simulink model "energybasedHosseinEd.old"  (R2020a)
settings: Solver=FixedStepDiscrete  StartTime=0.0  StopTime=Tsim  FixedStep=Ts  RelTol=1e-3
values from neighbouring files (symbols this model uses):
  EN_RATIO_LIMIT = param.EN_RATIO_LIMIT    [energybased.m]    (also in energybased.old.m = 0.3)
  En_Threshold = param.En_Threshold    [energybased.m]    (also in run.m = 2e-06; thresholdSet.m = 1e-08)
  M = ones(1,m)    [energybased.m]    (also in energybased.old.m; run.m)
  m = floor(m)    [energybased.m]    (also in energybased.old.m = ceil(Freq_stop0/Test.TPE)*Test.TPE/fT-m1; run.m)
  m1 = ceil(Freq_start0/fT)    [energybased.m]    (also in energybased.old.m)
  n_tpe = param.n_tpe    [energybased.m]    (also in energybased.old.m = 20; run.m = echdParam.n_tpe)
  nd_mean = round((1/Test.SF)/Ts)    [energybased.m]    (also in energybased.old.m; run.m = round((1/samplingFreq)/samplingInterval))
  num_delay = round((1/Test.SF)/Ts/2) * 5    [energybased.m]    (also in energybased.old.m; run.m = round((1/samplingFreq)/samplingInterval/2) * 5)
  TP_P0 = 1e1*eye(2*n_tpe)    [energybased.m]    (also in energybased.old.m; run.m)
  TP_PHI = zeros(2*n_tpe, 1)    [energybased.m]    (also in energybased.old.m; run.m)
  TP_Q = TP_R*lambda    [energybased.m]    (also in energybased.old.m; run.m)
  TP_q0 = zeros(2*n_tpe, 1)    [energybased.m]    (also in energybased.old.m; run.m)
  TP_R = 8.539750000056574E-6    (= 8.53975000006e-06)    [energybased.m]    (also in energybased.old.m; run.m)
  Ts = 1/properties.sampling    [energybased.m]    (also in energybased.old.m = 1/sampling)
  w_BOL = 1    [energybased.m]    (also in run.m; thresholdSet.m)
undefined symbols (not defined in the file or in its folder): Test
libraries: simulink x1
settings Model: Creator=Yudi Wang  LastModifiedBy=mhoss
settings DataIOCC: ReturnWorkspaceOutputs=off
settings DebuggingCC: ReadBeforeWriteMsg=DisableAll  WriteAfterWriteMsg=DisableAll  WriteAfterReadMsg=DisableAll  MultiTaskDSMMsg=none  ArithmeticOperatorsInVariantConditions=warning
settings ModelReferenceCC: UpdateModelReferenceTargets=IfOutOfDate
settings SFSimCC: SFSimEcho=off  SimUseLocalCustomCode=off  CustomCodeUndefinedFunction=UseInterfaceOnly
settings RTWCC: RTWUseLocalCustomCode=off

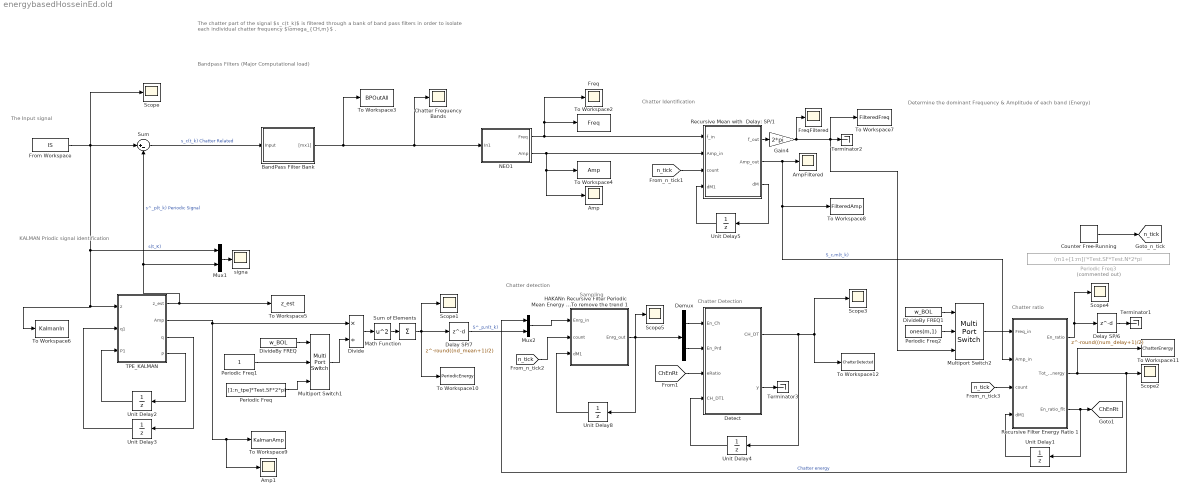
== system energybasedHosseinEd.old ==
  note: The chatter part of the signal $s_c(t_k)$ is filtered through a bank of band pass filters in order to isolate each individual chatter frequency $\omega_{CH,m}$ .
  note: Chatter Identification
  note: Chatter Detection
  note: Bandpass Filters
      | (Major Computational load)
  note: KALMAN
      | Priodic signal identification
  note: Chatter detection
  note: Chatter ratio
  note: The Input signal
  note: Determine the dominant Frequency & Amplitude of each band
      | (Energy)
  note: Sampling
  Amp : Scope
  Amp1 : Scope
  AmpFiltered : Scope
  BandPass Filter Bank : Subsystem
  Chatter Frequency Bands : Scope
  Counter Free-Running : simulink/Sources/Counter Free-Running  NumBits=32  tsamp=Ts
  Delay SP/6 : Delay  DelayLength=round((num_delay+1)/2)
  Delay SP/7 : Delay  DelayLength=round((nd_mean+1)/2)
  Demux : Demux  Outputs=2
  Detect : MATLAB Function  TreatAsAtomicUnit=on
  Divide : Product  Inputs=*/
  DivideBy FREQ : Constant  Value=w_BOL
  DivideBy FREQ1 : Constant  Value=w_BOL
  Freq : Scope
  FreqFiltered : Scope
  From Workspace : FromWorkspace  VariableName=IS  SampleTime=Ts  OutputAfterFinalValue=Setting to zero
  Gain4 : Gain  Gain=2*pi
  HAKANn Recursive Filter Periodic Mean Energy To remove the trend 1 : MATLAB Function  TreatAsAtomicUnit=on
  Math Function : Math  Operator=square  SignedPower=on  SaturateOnIntegerOverflow=on
  Multiport Switch1 : MultiPortSwitch  Inputs=2
  Multiport Switch2 : MultiPortSwitch  Inputs=2
  Mux1 : Mux  Inputs=2
  Mux2 : Mux  Inputs=2
  NEO1 : Subsystem
  Periodic Freq : Constant  Value=[1:n_tpe]*Test.SF*2*pi
  Periodic Freq1 : Constant
  Periodic Freq2 : Constant  Value=ones(m,1)
  Periodic Freq3 : Constant  Commented=on  Value=(m1+[1:m])'*Test.SF*Test.N*2*pi
  Recursive Mean with  Delay: SP/1 : MATLAB Function  TreatAsAtomicUnit=on
  Recursive Filter Energy Ratio 1 : MATLAB Function  TreatAsAtomicUnit=on
  Scope{,1..5} (6 alike) : Scope
  Sum : Sum  Inputs=|+-
  Sum of Elements : Sum  Inputs=+
  TPE_KALMAN : MATLAB Function  TreatAsAtomicUnit=on
  Terminator1 : Terminator
  Terminator2 : Terminator
  Terminator3 : Terminator
  To Workspace10 : ToWorkspace  VariableName=PeriodicEnergy  SaveFormat=Structure With Time  SampleTime=-1
  To Workspace11 : ToWorkspace  VariableName=ChatterEnergy  SaveFormat=Structure With Time  SampleTime=-1
  To Workspace12 : ToWorkspace  VariableName=ChatterDetected  SaveFormat=Structure With Time  SampleTime=-1
  To Workspace2 : ToWorkspace  VariableName=Freq  SaveFormat=Structure With Time  SampleTime=-1
  To Workspace3 : ToWorkspace  VariableName=BPOutAll  SaveFormat=Structure With Time  SampleTime=-1
  To Workspace4 : ToWorkspace  VariableName=Amp  SaveFormat=Structure With Time  SampleTime=-1
  To Workspace5 : ToWorkspace  VariableName=z_est  SaveFormat=Structure With Time  SampleTime=-1
  To Workspace6 : ToWorkspace  VariableName=KalmanIn  SaveFormat=Structure With Time  SampleTime=-1
  To Workspace7 : ToWorkspace  VariableName=FilteredFreq  SaveFormat=Structure With Time  SampleTime=-1
  To Workspace8 : ToWorkspace  VariableName=FilteredAmp  SaveFormat=Structure With Time  SampleTime=-1
  To Workspace9 : ToWorkspace  VariableName=KalmanAmp  SaveFormat=Structure With Time  SampleTime=-1
  Unit Delay1 : UnitDelay  SampleTime=Ts  HasFrameUpgradeWarning=on
  Unit Delay2 : UnitDelay  InitialCondition=TP_P0  SampleTime=-1  HasFrameUpgradeWarning=on
  Unit Delay3 : UnitDelay  InitialCondition=TP_q0  SampleTime=-1  HasFrameUpgradeWarning=on
  Unit Delay4 : UnitDelay  SampleTime=-1  HasFrameUpgradeWarning=on
  Unit Delay5 : UnitDelay  SampleTime=-1  HasFrameUpgradeWarning=on
  Unit Delay8 : UnitDelay  SampleTime=Ts  HasFrameUpgradeWarning=on
  signa : Scope
  tag scope: ChEnRt=global, n_tick=global
  wires:
  Mux1/1 -> signa/1
  HAKANn Recursive Filter Periodic Mean Energy To remove the trend 1/1(Enrg_out) -> Demux/1, Scope5/1, Unit Delay8/1
  Sum/1 -> BandPass Filter Bank/1(Input)  "s_c(t_k) Chatter Related"
  Multiport Switch2/1 -> Recursive Filter Energy Ratio 1/1(Freq_in)
  Periodic Freq1/1 -> Multiport Switch1/2
  TPE_KALMAN/1(z_est) -> Mux1/2, Sum/2, To Workspace5/1  "s^_p(t_k) Periodic Signal"
  Math Function/1 -> Sum of Elements/1
  TPE_KALMAN/4(P) -> Unit Delay2/1
  BandPass Filter Bank/1("[mx1]") -> To Workspace3/1, NEO1/1(In1), Chatter Frequency Bands/1
  Detect/2(y) -> Terminator3/1
  [n_tick] -> HAKANn Recursive Filter Periodic Mean Energy To remove the trend 1/2(count)
  TPE_KALMAN/2(Amp) -> Divide/1, Amp1/1, To Workspace9/1
  Counter Free-Running/1 -> [n_tick]
  NEO1/1(Freq) -> Recursive Mean with  Delay: SP/1/1(f_in), Freq/1, To Workspace2/1
  Recursive Filter Energy Ratio 1/3(En_ratio_flt) -> [ChEnRt], Unit Delay1/1
  Detect/1(CH_DT) -> Unit Delay4/1, To Workspace12/1, Scope3/1
  [n_tick] -> Recursive Mean with  Delay: SP/1/3(count)
  Recursive Filter Energy Ratio 1/2(Tot_CH_Energy) -> To Workspace11/1, Mux2/1, Scope2/1  "Chatter energy"
  Periodic Freq2/1 -> Multiport Switch2/2
  Recursive Mean with  Delay: SP/1/3(dM) -> Unit Delay5/1
  Unit Delay4/1 -> Detect/4(CH_DT1)
  Recursive Mean with  Delay: SP/1/1(f_out) -> Gain4/1
  Divide/1 -> Math Function/1
  NEO1/2(Amp) -> Recursive Mean with  Delay: SP/1/2(Amp_in), Amp/1, To Workspace4/1
  Periodic Freq/1 -> Multiport Switch1/3
  From Workspace/1 -> Scope/1, To Workspace6/1, TPE_KALMAN/1(z), Mux1/1, Sum/1  "s(t_K)"
  Unit Delay8/1 -> HAKANn Recursive Filter Periodic Mean Energy To remove the trend 1/3(dM1)
  Unit Delay5/1 -> Recursive Mean with  Delay: SP/1/4(dM1)
  [n_tick] -> Recursive Filter Energy Ratio 1/3(count)
  Demux/2 -> Detect/2(En_Prd)
  TPE_KALMAN/3(q) -> Unit Delay3/1
  DivideBy FREQ/1 -> Multiport Switch1/1
  Unit Delay1/1 -> Recursive Filter Energy Ratio 1/4(dM1)
  Gain4/1 -> FreqFiltered/1, Terminator2/1, To Workspace7/1, Multiport Switch2/3
  Multiport Switch1/1 -> Divide/2
  Recursive Filter Energy Ratio 1/1(En_ratio) -> Delay SP/6/1, Scope4/1
  Demux/1 -> Detect/1(En_Ch)
  [ChEnRt] -> Detect/3(eRatio)
  Unit Delay3/1 -> TPE_KALMAN/2(q1)
  Unit Delay2/1 -> TPE_KALMAN/3(P1)
  Mux2/1 -> HAKANn Recursive Filter Periodic Mean Energy To remove the trend 1/1(Enrg_in)
  Sum of Elements/1 -> To Workspace10/1, Delay SP/7/1, Scope1/1
  DivideBy FREQ1/1 -> Multiport Switch2/1
  Recursive Mean with  Delay: SP/1/2(Amp_out) -> Recursive Filter Energy Ratio 1/2(Amp_in), To Workspace8/1, AmpFiltered/1  "S_c,m(t_k)"
  Delay SP/6/1 -> Terminator1/1
  Delay SP/7/1 -> Mux2/2  "S^_p,n(t_k)"

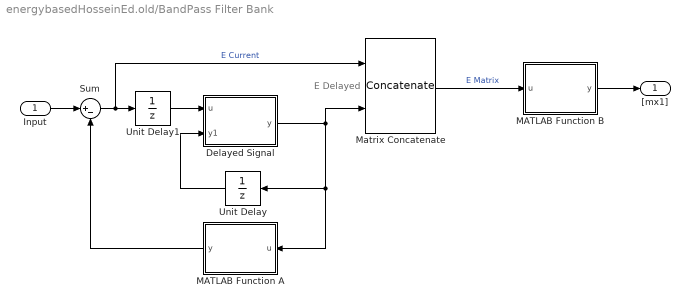
== system energybasedHosseinEd.old/BandPass Filter Bank ==
  note: E Delayed
  Input : Inport
  Delayed Signal : MATLAB Function  TreatAsAtomicUnit=on
  MATLAB Function A : MATLAB Function  TreatAsAtomicUnit=on
  MATLAB Function B : MATLAB Function  TreatAsAtomicUnit=on
  Matrix Concatenate : Concatenate  Mode=Multidimensional array  ConcatenateDimension=2
  Sum : Sum  Inputs=|+-
  Unit Delay : UnitDelay  SampleTime=-1  HasFrameUpgradeWarning=on
  Unit Delay1 : UnitDelay  SampleTime=-1  HasFrameUpgradeWarning=on
  "[mx1]" : Outport  VectorParamsAs1DForOutWhenUnconnected=off
  wires:
  Delayed Signal/1(y) -> Unit Delay/1, MATLAB Function A/1(u), Matrix Concatenate/2
  Unit Delay/1 -> Delayed Signal/2(y1)
  Unit Delay1/1 -> Delayed Signal/1(u)
  Sum/1 -> Unit Delay1/1, Matrix Concatenate/1  "E Current"
  Input/1 -> Sum/1
  MATLAB Function A/1(y) -> Sum/2
  Matrix Concatenate/1 -> MATLAB Function B/1(u)  "E Matrix"
  MATLAB Function B/1(y) -> "[mx1]"/1

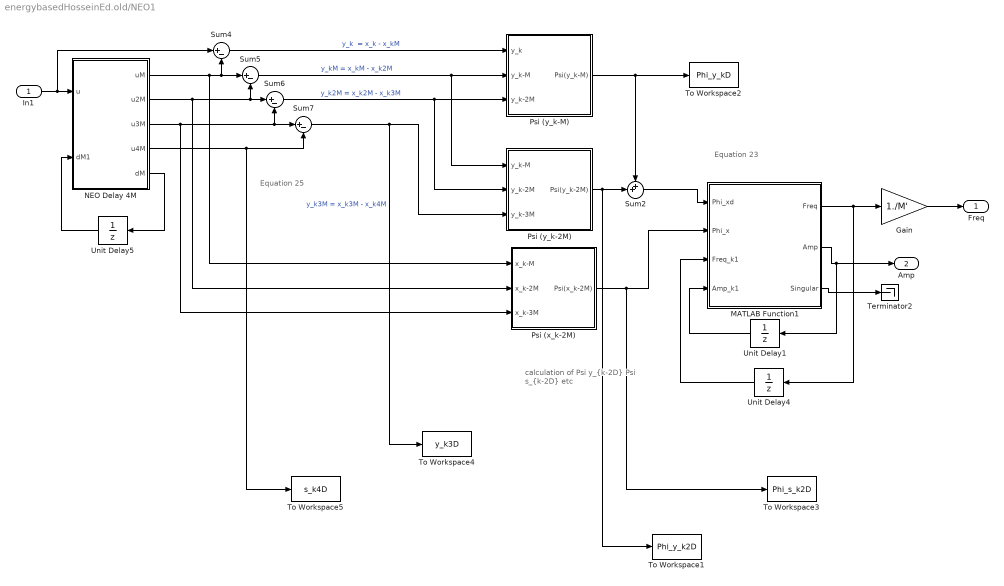
== system energybasedHosseinEd.old/NEO1 ==
  note: calculation of
      | Psi y_{k-2D}
      | Psi s_{k-2D} etc
  note: Equation 23
  note: Equation 25
  In1 : Inport
  Gain : Gain  Gain=1./M'
  MATLAB Function1 : MATLAB Function  TreatAsAtomicUnit=on
  NEO Delay 4M : MATLAB Function  TreatAsAtomicUnit=on
  Psi (x_k-2M) : Subsystem
  Psi (y_k-2M) : Subsystem
  Psi (y_k-M) : Subsystem
  Sum2 : Sum  Inputs=++|
  Sum{4..7} (4 alike) : Sum  Inputs=|+-
  Terminator2 : Terminator
  To Workspace1 : ToWorkspace  VariableName=Phi_y_k2D  SaveFormat=Structure With Time  SampleTime=-1
  To Workspace2 : ToWorkspace  VariableName=Phi_y_kD  SaveFormat=Structure With Time  SampleTime=-1
  To Workspace3 : ToWorkspace  VariableName=Phi_s_k2D  SaveFormat=Structure With Time  SampleTime=-1
  To Workspace4 : ToWorkspace  VariableName=y_k3D  SaveFormat=Structure With Time  SampleTime=-1
  To Workspace5 : ToWorkspace  VariableName=s_k4D  SaveFormat=Structure With Time  SampleTime=-1
  Unit Delay1 : UnitDelay  SampleTime=Ts  HasFrameUpgradeWarning=on
  Unit Delay4 : UnitDelay  SampleTime=Ts  HasFrameUpgradeWarning=on
  Unit Delay5 : UnitDelay  SampleTime=Ts  HasFrameUpgradeWarning=on
  Freq : Outport  VectorParamsAs1DForOutWhenUnconnected=off
  Amp : Outport  Port=2  VectorParamsAs1DForOutWhenUnconnected=off
  wires:
  Sum4/1 -> Psi (y_k-M)/1(y_k)  "y_k  = x_k - x_kM"
  NEO Delay 4M/5(dM) -> Unit Delay5/1
  Unit Delay5/1 -> NEO Delay 4M/2(dM1)
  NEO Delay 4M/1(uM) -> Sum4/2, Sum5/1, Psi (x_k-2M)/1(x_k-M)
  Sum5/1 -> Psi (y_k-M)/2(y_k-M), Psi (y_k-2M)/1(y_k-M)  "y_kM = x_kM - x_k2M"
  NEO Delay 4M/3(u3M) -> Sum6/2, Sum7/1, Psi (x_k-2M)/3(x_k-3M)
  Sum6/1 -> Psi (y_k-M)/3(y_k-2M), Psi (y_k-2M)/2(y_k-2M)  "y_k2M = x_k2M - x_k3M"
  In1/1 -> NEO Delay 4M/1(u), Sum4/1
  Psi (y_k-M)/1(Psi(y_k-M)) -> To Workspace2/1, Sum2/1
  NEO Delay 4M/2(u2M) -> Sum6/1, Sum5/2, Psi (x_k-2M)/2(x_k-2M)
  NEO Delay 4M/4(u4M) -> To Workspace5/1, Sum7/2
  Sum7/1 -> To Workspace4/1, Psi (y_k-2M)/3(y_k-3M)  "y_k3M = x_k3M - x_k4M"
  Psi (y_k-2M)/1(Psi(y_k-2M)) -> To Workspace1/1, Sum2/2
  Unit Delay1/1 -> MATLAB Function1/4(Amp_k1)
  Unit Delay4/1 -> MATLAB Function1/3(Freq_k1)
  MATLAB Function1/1(Freq) -> Unit Delay4/1, Gain/1
  Gain/1 -> Freq/1
  MATLAB Function1/2(Amp) -> Unit Delay1/1, Amp/1
  Psi (x_k-2M)/1(Psi(x_k-2M)) -> To Workspace3/1, MATLAB Function1/2(Phi_x)
  Sum2/1 -> MATLAB Function1/1(Phi_xd)
  MATLAB Function1/3(Singular) -> Terminator2/1

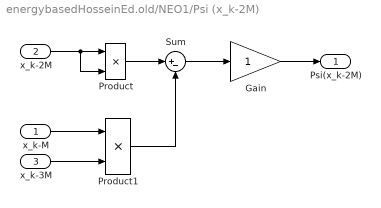
== system energybasedHosseinEd.old/NEO1/Psi (x_k-2M) ==
  x_k-M : Inport
  x_k-2M : Inport  Port=2
  x_k-3M : Inport  Port=3
  Gain : Gain
  Product : Product
  Product1 : Product
  Sum : Sum  Inputs=|+-
  Psi(x_k-2M) : Outport  VectorParamsAs1DForOutWhenUnconnected=off
  wires:
  Product1/1 -> Sum/2
  Sum/1 -> Gain/1
  Gain/1 -> Psi(x_k-2M)/1
  x_k-M/1 -> Product1/1
  x_k-3M/1 -> Product1/2
  Product/1 -> Sum/1
  x_k-2M/1 -> Product/2, Product/1

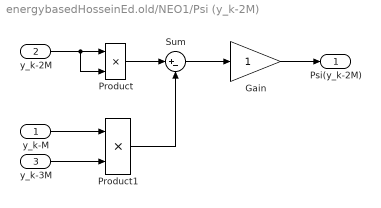
== system energybasedHosseinEd.old/NEO1/Psi (y_k-2M) ==
  y_k-M : Inport
  y_k-2M : Inport  Port=2
  y_k-3M : Inport  Port=3
  Gain : Gain
  Product : Product
  Product1 : Product
  Sum : Sum  Inputs=|+-
  Psi(y_k-2M) : Outport  VectorParamsAs1DForOutWhenUnconnected=off
  wires:
  y_k-2M/1 -> Product/1, Product/2
  Product/1 -> Sum/1
  y_k-3M/1 -> Product1/2
  y_k-M/1 -> Product1/1
  Gain/1 -> Psi(y_k-2M)/1
  Sum/1 -> Gain/1
  Product1/1 -> Sum/2

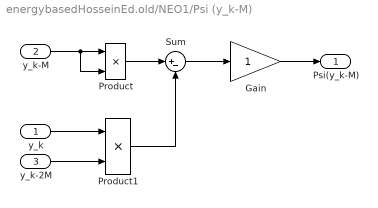
== system energybasedHosseinEd.old/NEO1/Psi (y_k-M) ==
  y_k : Inport
  y_k-M : Inport  Port=2
  y_k-2M : Inport  Port=3
  Gain : Gain
  Product : Product
  Product1 : Product
  Sum : Sum  Inputs=|+-
  Psi(y_k-M) : Outport  VectorParamsAs1DForOutWhenUnconnected=off
  wires:
  Product1/1 -> Sum/2
  Sum/1 -> Gain/1
  Gain/1 -> Psi(y_k-M)/1
  y_k/1 -> Product1/1
  y_k-2M/1 -> Product1/2
  Product/1 -> Sum/1
  y_k-M/1 -> Product/2, Product/1

== matlab function energybasedHosseinEd.old/Detect ==
  settings: updateMethod=DISCRETE  sampleTime=Ts
  data: CH_DT output size=[1,1]; y output size=[3,1]; En_Ch input size=[1,1]; En_Prd input size=[1,1]; eRatio input size=[m, 1]; CH_DT1 input; En_Threshold parameter; EN_RATIO_LIMIT parameter
function [CH_DT, y]= fcn(En_Ch, En_Prd, eRatio, CH_DT1, En_Threshold, EN_RATIO_LIMIT)

% CH_DT=0;
EnergyRatio = En_Ch/(En_Ch+En_Prd);
y=[1;1;1];

if CH_DT1==0 && EnergyRatio>0.5  % entry
    CH_DT=0; % keep detect variable zero
elseif CH_DT1==1 && EnergyRatio>0.1 % chatter continuing
    CH_DT=1;% do nothing
    [B,I]=sort(eRatio,'descend');
    y = I(1:3);
% elseif EnergyRatio>EN_RATIO_LIMIT && StdRatio>STD_RATIO_LIMIT && En_Prd>En_Threshold
elseif EnergyRatio>EN_RATIO_LIMIT && En_Prd>En_Threshold
    CH_DT=1;
    [B,I]=sort(eRatio,'descend');
    y = I(1:3);
elseif EnergyRatio<0.1 % no chatter, stable
    CH_DT=0;
else
    CH_DT=0;
end


y=sort(y);

== matlab function energybasedHosseinEd.old/Recursive Mean with  Delay: SP//1 ==
  settings: updateMethod=DISCRETE  sampleTime=Ts
  data: f_in input size=[m,1]; Amp_in input size=[m,1]; count input; f_out output size=[m, 1]; Amp_out output size=[m,1]; dM1 input size=[2*m, 1]; dM output size=[2*m, 1]; m parameter size=1; nd_mean parameter size=1
function [f_out, Amp_out, dM] = fcn(f_in, Amp_in, count, dM1, m, nd_mean)


if count < nd_mean
    j = double(count);
    if count == 0
        f_out = zeros(m,1);
        Amp_out = zeros(m,1);
    else
    f_out = (j-1)/j*dM1(1:m,1)+1/j*f_in;
    Amp_out = (j-1)/j*dM1(m+1:end,1)+1/j*Amp_in;
    end
else
    f_out = (nd_mean-1)/nd_mean*dM1(1:m,1)+1/nd_mean*f_in;
    Amp_out = (nd_mean-1)/nd_mean*dM1(m+1:end,1)+1/nd_mean*Amp_in;
end




% -----------------------------------------------------------
dM=[f_out; Amp_out];

== matlab function energybasedHosseinEd.old/HAKANn Recursive Filter Periodic Mean Energy To remove the trend 1 ==
  settings: updateMethod=DISCRETE  sampleTime=Ts
  data: Enrg_in input size=[2,1]; count input; Enrg_out output size=[2,1]; dM1 input size=[2,1]; num_delay parameter size=1
function Enrg_out  = fcn(Enrg_in, count, dM1, num_delay)
%#codegen


m=length(Enrg_in);
if count < num_delay
    j=double(count);
    if count ==0
        Enrg_out =zeros(m,1);
    else
        Enrg_out=(j-1)/j*dM1+1/j*Enrg_in;
    end
else
    Enrg_out=(num_delay-1)/num_delay*dM1+1/num_delay*Enrg_in;
end

== matlab function energybasedHosseinEd.old/TPE_KALMAN ==
  settings: updateMethod=DISCRETE  sampleTime=Ts
  data: z input size=1; z_est output size=1; Amp output size=[n_tpe 1]; q1 input size=[2*n_tpe, 1]; P1 input size=[2*n_tpe, 2*n_tpe]; TP_Q parameter size=1; TP_R parameter size=1; TP_PHI parameter size=[2*n_tpe, 1]; q output size=[2*n_tpe, 1]; P output size=[2*n_tpe, 2*n_tpe]
function [z_est, Amp, q, P] = fcn(z, q1, P1, TP_Q, TP_R, TP_PHI)
n_tpe = round(length(q1)/2);
%n_tpe = 20;
Amp=zeros(n_tpe, 1);
q_hat_pro = zeros(2*n_tpe, 1);
P_pro = zeros(2*n_tpe, 2*n_tpe);
K = zeros(2*n_tpe, 1);
q = zeros(2*n_tpe, 1);
P = zeros(2*n_tpe, 2*n_tpe);

%   PRIORI ESTIMATE
%q_hat_pro = TP_PHI * q1;
%P_pro = TP_PHI*P1*TP_PHI'+TP_Q;
for i = 0:n_tpe-1
    q_hat_pro(2*i+1) = TP_PHI(2*i+1)*q1(2*i+1)-TP_PHI(2*i+1+1)*q1(2*i+1+1);
    q_hat_pro(2*i+1+1) = TP_PHI(2*i+1+1)*q1(2*i+1)+TP_PHI(2*i+1)*q1(2*i+1+1);
end

for i = 0:n_tpe-1
    for j = 0:n_tpe-1
        P_pro(2*i+1, 2*j+1) = TP_PHI(2*j+1)*(P1(2*i+1,2*j+1)*TP_PHI(2*i+1) - P1(2*i+1+1, 2*j+1)*TP_PHI(2*i+1+1))-...
                              TP_PHI(2*j+1+1)*(P1(2*i+1,2*j+1+1)*TP_PHI(2*i+1) - P1(2*i+1+1,2*j+1+1)*TP_PHI(2*i+1+1));
        P_pro(2*i+1, 2*j+1+1) = TP_PHI(2*j+1+1)*(P1(2*i+1,2*j+1)*TP_PHI(2*i+1) - P1(2*i+1+1, 2*j+1)*TP_PHI(2*i+1+1))+...
                                TP_PHI(2*j+1)*(P1(2*i+1,2*j+1+1)*TP_PHI(2*i+1) - P1(2*i+1+1,2*j+1+1)*TP_PHI(2*i+1+1));
        P_pro(2*i+1+1, 2*j+1) = TP_PHI(2*j+1)*(P1(2*i+1,2*j+1)*TP_PHI(2*i+1+1) + P1(2*i+1+1, 2*j+1)*TP_PHI(2*i+1))-...
                                TP_PHI(2*j+1+1)*(P1(2*i+1,2*j+1+1)*TP_PHI(2*i+1+1) + P1(2*i+1+1,2*j+1+1)*TP_PHI(2*i+1));
        P_pro(2*i+1+1, 2*j+1+1) = TP_PHI(2*j+1+1)*(P1(2*i+1,2*j+1)*TP_PHI(2*i+1+1) + P1(2*i+1+1, 2*j+1)*TP_PHI(2*i+1))+...
                                  TP_PHI(2*j+1)*(P1(2*i+1,2*j+1+1)*TP_PHI(2*i+1+1) + P1(2*i+1+1,2*j+1+1)*TP_PHI(2*i+1));
    end
end

for i = 0:2*n_tpe-1
    P_pro(i+1,i+1) = P_pro(i+1,i+1) + TP_Q;
end

%   POSTERIORI ESTIMATE
%K = P_pro*TP_H'*(TP_H*P_pro*TP_H' + TP_R)^-1;
invSum = 0;
for i = 0:n_tpe-1
    for j = 0:n_tpe-1
        invSum = invSum + P_pro(2*i+1,2*j+1);
    end
end

inverse = 1.0/(invSum + TP_R);
for i = 0 : 2*n_tpe-1
    tempSum = 0;
    for j = 0:n_tpe-1
        tempSum = tempSum + P_pro(i+1, 2*j+1);        
    end
    K(i+1) = inverse*tempSum;
end

%q = q_hat_pro + K*(z - TP_H*q_hat_pro);
sMinusHqk = z;
for i = 0:n_tpe-1
    sMinusHqk = sMinusHqk - q_hat_pro(2*i+1);
end

for i = 0:2*n_tpe-1
    q(i+1) = q_hat_pro(i+1)+K(i+1)*sMinusHqk;
end
    
%P = (eye(2*n_tpe)-K*TP_H)*P_pro;
for j = 0:2*n_tpe-1
    tempSum = 0;
    for k = 0:n_tpe-1
        tempSum = tempSum + P_pro(2*k+1,j+1);
    end
    
    for i = 0:2*n_tpe-1
        P(i+1,j+1) = -K(i+1)*tempSum+P_pro(i+1,j+1);
    end
end

%z_est = TP_H*q;
z_est = 0;
for i = 0:n_tpe-1
    z_est = z_est + q(2*i+1);
end

for j=1:n_tpe
    Amp(j,1) = sqrt(q(2*j-1)^2 + q(2*j)^2);
end

%% 
% 
% for i = 0:n_tpe-1
%     q_hat_pro(2*i+1) = TP_PHI(2*i+1)*q1(2*i+1)-TP_PHI(2*i+1+1)*q1(2*i+1+1);
%     q_hat_pro(2*i+1+1) = TP_PHI(2*i+1+1)*q1(2*i+1)-TP_PHI(2*i+1)*q1(2*i+1+1);
% end
% 
% for i = 0:n_tpe-1
%     for j = 0:n_tpe-1
%         P_pro(2*i+1, 2*j+1) = TP_PHI(2*j+1)*P1(2*i+1,2*j+1)*TP_PHI(2*i+1) - P1(2*i+1+1, 2*j+1)*TP_PHI(2*i+1+1)-TP_PHI(2*j+1+1)*P1(2*i+1,2*j+1+1)*TP_PHI(2*i+1) - P1(2*i+1+1,2*j+1+1)*TP_PHI(2*i+1+1);
%         P_pro(2*i+1, 2*j+1+1) = TP_PHI(2*j+1+1)*P1(2*i+1,2*j+1)*TP_PHI(2*i+1) - P1(2*i+1+1, 2*j+1)*TP_PHI(2*i+1+1)+TP_PHI(2*j+1)*P1(2*i+1,2*j+1+1)*TP_PHI(2*i+1) - P1(2*i+1+1,2*j+1+1)*TP_PHI(2*i+1+1);
%         P_pro(2*i+1, 2*j) = TP_PHI(2*j)*P1(2*i,2*j)*TP_PHI(2*i+1) + P1(2*i+1, 2*j)*TP_PHI(2*i)-TP_PHI(2*j+1)*P1(2*i,2*j+1)*TP_PHI(2*i+1) + P1(2*i+1,2*j+1)*TP_PHI(2*i);
%         P_pro(2*i+1, 2*j+1) = TP_PHI(2*j+1)*P1(2*i,2*j)*TP_PHI(2*i+1) + P1(2*i+1, 2*j)*TP_PHI(2*i)+TP_PHI(2*j)*P1(2*i,2*j+1)*TP_PHI(2*i+1) + P1(2*i+1,2*j+1)*TP_PHI(2*i);
%     end
% end
% 
% for i = 1:2*n_tpe
%     P_pro(i,i) = P_pro(i,i) + TP_Q;
% end
% 
% %   POSTERIORI ESTIMATE
% %K = P_pro*TP_H'*(TP_H*P_pro*TP_H' + TP_R)^-1;
% for i = 1:n_tpe
%     for j = 1:n_tpe
%         invSum = invSum + P_pro(2*i,2*j);
%     end
% end
% 
% inverse = 1.0/(invSum + TP_R);
% for i = 1 : 2*n_tpe
%     tempSum = 0;
%     for j = 1:n_tpe
%         tempSum = tempSum + P_pro(i, 2*j);        
%     end
%     K(i) = inverse*tempSum;
% end
% 
% %q = q_hat_pro + K*(z - TP_H*q_hat_pro);
% sMinusHqk = z;
% for i = 1:n_tpe
%     sMinusHqk = sMinusHqk - q_hat_pro(2*i);
% end
% 
% for i = 1:2*n_tpe
%     q(i) = q_hat_pro(i)+K(i)*sMinusHqk;
% end
%     
% %P = (eye(2*n_tpe)-K*TP_H)*P_pro;
% for j = 1:2*n_tpe
%     tempSum = 0;
%     for k = 1:n_tpe
%         tempSum = tempSum + P_pro(2*k,j);
%     end
%     
%     for i = 1:2*n_tpe
%         P(i,j) = -K(i)*tempSum*P_pro(i,j);
%     end
% end
% 
% %z_est = TP_H*q;
% z_est = 0;
% for i = 1:n_tpe
%     z_est = z_est + q(2*i);
% end
% 
% for j=1:n_tpe
%     Amp(j,1) = sqrt(q(2*j-1)^2 + q(2*j)^2);
% end
%

== matlab function energybasedHosseinEd.old/NEO1/MATLAB Function1 ==
  settings: updateMethod=DISCRETE  sampleTime=Ts
  data: Phi_xd input size=[m, 1]; Freq output size=[m,1]; Phi_x input size=[m, 1]; Ts parameter size=1; Freq_k1 input size=[m,1]; Amp_k1 input size=[m,1]; Amp output size=[m,1]; Singular output size=1; m parameter size=1
function [Freq,Amp, Singular] = fcn(Phi_xd, Phi_x, Ts, Freq_k1, Amp_k1, m)
% m = length(Phi_x);
% Freq=zeros(m,1);
% Amp =zeros(m,1);

Freq = Freq_k1;
Amp = Amp_k1;

%% Add to eliminate the FIND command
for i=1:m
    if (Phi_x(i) >0 && Phi_xd(i) >0 && Phi_xd(i)<8*Phi_x(i))
        index=i;
        dum = 1-Phi_xd(index)./Phi_x(index)/4;
        Freq(index) = acos(dum)/2/pi/Ts; % Hz
        Amp(index) = sqrt(Phi_x(index)./(1-dum.^2));
        Singular=0;%    FOR MONITORING CNA BE DELERTED
    else
        Singular=1;
    end
end

end

== matlab function energybasedHosseinEd.old/NEO1/NEO Delay 4M ==
  settings: updateMethod=DISCRETE  sampleTime=Ts
  data: u input size=[m,1]; uM output size=[m, 1]; u2M output size=[m, 1]; u3M output size=[m, 1]; u4M output size=[m, 1]; M parameter size=[1, m]; dM1 input size=[m, 4*nd+1]; dM output size=[m, 4*nd+1]; m parameter size=1
function [uM,u2M, u3M, u4M, dM] = fcn(u, M, dM1, m)
%#codegen
uM=zeros(m,1);
u2M=zeros(m,1);
u3M=zeros(m,1);
u4M=zeros(m,1);


nd=max(M);
dM=[u,dM1(:,1:4*nd)];

for i=1:m
    uM(i,1)= dM(i,M(i)+1)';
    u2M(i,1)=dM(i,2*M(i)+1)';
    u3M(i,1)=dM(i,3*M(i)+1)';
    u4M(i,1)=dM(i,4*M(i)+1)';
end

== matlab function energybasedHosseinEd.old/BandPass Filter Bank/Delayed Signal ==
  settings: updateMethod=DISCRETE  sampleTime=Ts
  data: u input size=[m, 1]; y output size=[m, 2*n]; y1 input size=[m, 2*n]
function y = fcn(u, y1)
%   u: [m,1] [12,1]
%   y: [m,2n] [12,8]
Nd = size(y1,2);

y = [u,y1(:,1:Nd-1)]; %[12,8]

== matlab function energybasedHosseinEd.old/BandPass Filter Bank/MATLAB Function A ==
  settings: updateMethod=DISCRETE  sampleTime=Ts
  data: u input size=[m, 2*n]; y output size=[m,1]; A parameter size=[m, 2*n]
function y = fcn(u, A)
m = size(A,1);
y = zeros(m,1); %[12 x 1]
for i=1:m
    y(i) = A(i,:)*u(i,:)'; % [1 x 8]*[8*1]
end

== matlab function energybasedHosseinEd.old/BandPass Filter Bank/MATLAB Function B ==
  settings: updateMethod=DISCRETE  sampleTime=Ts
  data: u input size=[m, 2*n+1]; y output size=[m,1]; B parameter size=[m, 2*n+1]
function y = fcn(u, B)
m = size(B,1); %12
y = zeros(m,1); %[m x 1]
for i=1:m
    y(i) = B(i,:)*u(i,:)';
end

== matlab function energybasedHosseinEd.old/Recursive Filter Energy Ratio 1 ==
  settings: updateMethod=DISCRETE  sampleTime=Ts
  data: Freq_in input size=[m,1]; Amp_in input size=[m, 1]; count input; En_ratio output size=[m,1]; Tot_CH_Energy output; En_ratio_flt output size=[m,1]; dM1 input size=[m,1]; num_delay parameter size=1
function [En_ratio, Tot_CH_Energy, En_ratio_flt] = fcn(Freq_in, Amp_in, count, dM1, num_delay)
%#codegen

m=length(Amp_in);
Energy=zeros(m,1);

for i=1:m
    if Freq_in(i)==0
        Energy(i,1) =0;
    else
        Energy(i,1) =(Amp_in(i,1)/Freq_in(i,1)).^2;
    end  
end
Tot_CH_Energy = sum(Energy);

if Tot_CH_Energy ==0
    En_ratio = zeros(m,1);
else
    En_ratio = Energy/Tot_CH_Energy ;
end

if count < num_delay
    j=double(count);
    if count ==0
        En_ratio_flt=zeros(m,1);
    else
      En_ratio_flt=(j-1)/j*dM1+1/j*En_ratio ;
    end
else
    En_ratio_flt=(num_delay-1)/num_delay*dM1+1/num_delay*En_ratio ;
end
